simulink model "p4"  (R2020b)
settings: Solver=ode15s  StartTime=0.0  StopTime=0.2  MaxStep=0.0001  RelTol=1e-3
values from neighbouring files (symbols this model uses):
  b = 3.5077E-6    (= 3.5077e-06)    [pid.m]    (also in pidcalculation.m)
  J = 3.2284E-6    (= 3.2284e-06)    [pid.m]    (also in pidcalculation.m)
  K = 0.0274    [pid.m]    (also in pidcalculation.m)
  L = 2.75E-6    (= 2.75e-06)    [pid.m]    (also in pidcalculation.m)
  R = 4    [pid.m]    (also in pidcalculation.m)
settings Model: Creator=WELCOME  LastModifiedBy=WELCOME

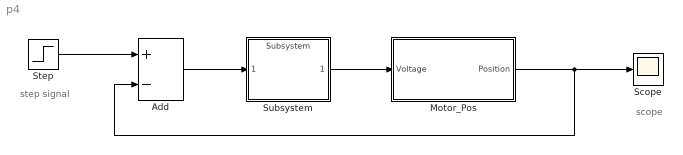
== system p4 ==
  note: scope
  note: step signal
  Add : Sum  Inputs=+-
  Motor_Pos : Subsystem
  Scope : Scope
  Step : Step  Time=0  SampleTime=0
  Subsystem : ModelReference  ModelNameDialog=Subsystem  SimulationMode=Normal  ModelReferenceVersion=1.7
  wires:
  Subsystem/1 -> Motor_Pos/1(Voltage)
  Motor_Pos/1(Position) -> Add/2, Scope/1
  Add/1 -> Subsystem/1
  Step/1 -> Add/1

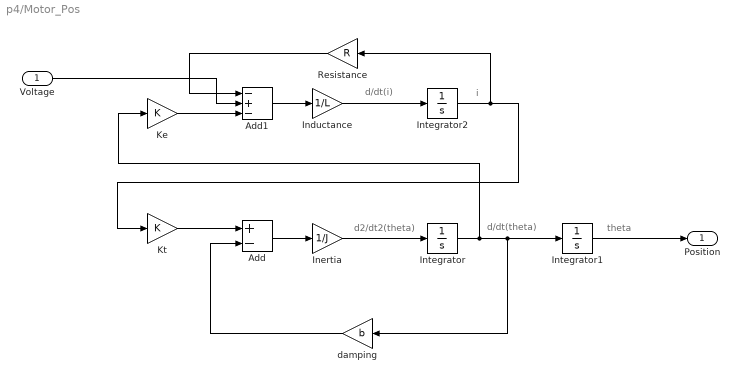
== system p4/Motor_Pos ==
  note: i
  note: d2/dt2(theta)
  note: d/dt(i)
  note: d/dt(theta)
  note: theta
  Voltage : Inport
  Add : Sum  Inputs=+-
  Add1 : Sum  Inputs=-+-
  Inductance : Gain  Gain=1/L
  Inertia : Gain  Gain=1/J
  Integrator : Integrator
  Integrator1 : Integrator
  Integrator2 : Integrator
  Ke : Gain  Gain=K
  Kt : Gain  Gain=K
  Resistance : Gain  Gain=R
  damping : Gain  Gain=b
  Position : Outport
  wires:
  Integrator2/1 -> Resistance/1, Kt/1
  Kt/1 -> Add/1
  damping/1 -> Add/2
  Voltage/1 -> Add1/2
  Integrator/1 -> Ke/1, damping/1, Integrator1/1
  Add1/1 -> Inductance/1
  Inductance/1 -> Integrator2/1
  Ke/1 -> Add1/3
  Add/1 -> Inertia/1
  Integrator1/1 -> Position/1
  Resistance/1 -> Add1/1
  Inertia/1 -> Integrator/1
